simulink model "simulink_yalmip"  (R2021b)
settings: Solver=VariableStepAuto  StartTime=0.0  StopTime=Tsim  FixedStep=Ts  RelTol=1e-3
values from neighbouring files (symbols this model uses):
  N = 10    [main.m]
  Ts = 0.01    [main.m]
  x0 = zeros(nx,1)    [main.m]
undefined symbols (not defined in the file or in its folder): A, B, C
settings Model: Creator=PBM  LastModifiedBy=PBM

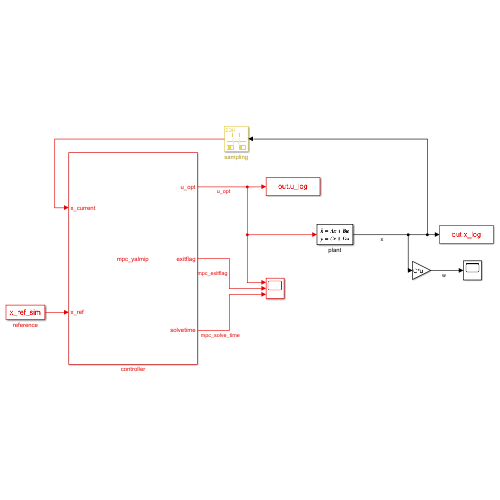
[thumbnail: Simulink's stored preview of the top-level diagram]
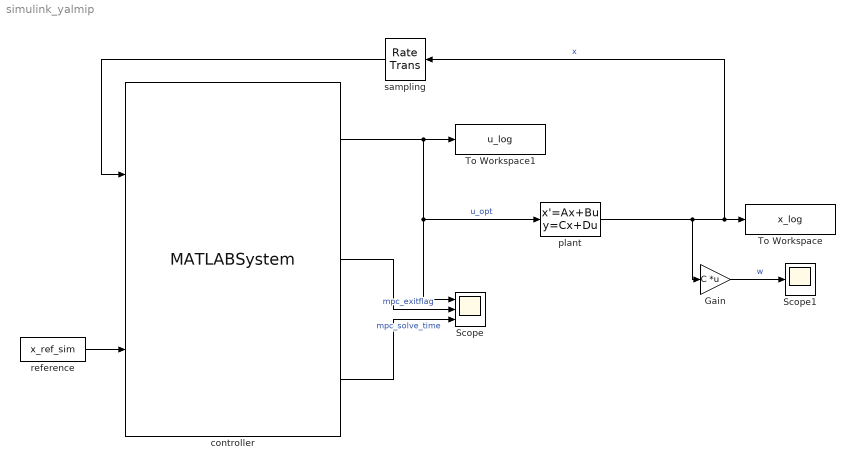
== system simulink_yalmip ==
  Gain : Gain  Gain=C  Multiplication=Matrix(K*u)
  Scope : Scope  NumInputPorts=3
  Scope1 : Scope
  To Workspace : ToWorkspace  VariableName=x_log  SampleTime=Ts
  To Workspace1 : ToWorkspace  VariableName=u_log  SampleTime=Ts
  controller : MATLABSystem  System=mpc_yalmip  Ts=Ts  nu=nu  N=N  SimulateUsing=Interpreted execution
      mask Type: mpc_yalmip
      mask Display:
      | disp('mpc_yalmip');
      | port_label('input',1,'x_current');
      | port_label('input',2,'x_ref');
      | port_label('output',1,'u_opt');
      | port_label('output',2,'exitflag');
      | port_label('output',3,'solvetime');
  plant : StateSpace  A=A  B=B  C="eye(nx)  % to get all states out of the block"  D=zeros(size(B))  InitialCondition=x0
  reference : FromWorkspace  VariableName=x_ref_sim  SampleTime=Ts
  sampling : RateTransition  InitialCondition=x0  OutPortSampleTime=Ts
  wires:
  plant/1 -> Gain/1, To Workspace/1, sampling/1  "x"
  reference/1 -> controller/2
  controller/1 -> To Workspace1/1, plant/1, Scope/1  "u_opt"
  controller/2 -> Scope/2  "mpc_exitflag"
  controller/3 -> Scope/3  "mpc_solve_time"
  Gain/1 -> Scope1/1  "w"
  sampling/1 -> controller/1
